simulink model "Product12"  (R2023a)
settings: Solver=VariableStepAuto  StartTime=0.0  StopTime=10.0  RelTol=1e-3
settings Model: Creator=Egypt_Laptop  LastModifiedBy=Egypt_Laptop

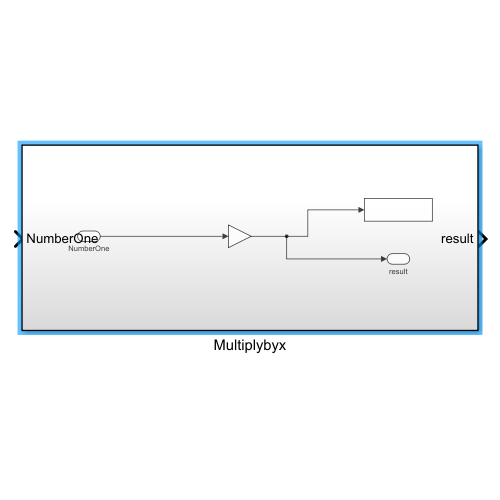
[thumbnail: Simulink's stored preview of the top-level diagram]
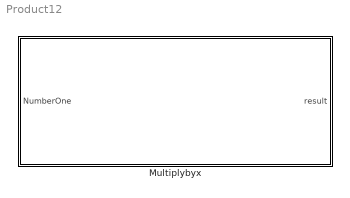
== system Product12 ==
  Multiplybyx : Subsystem

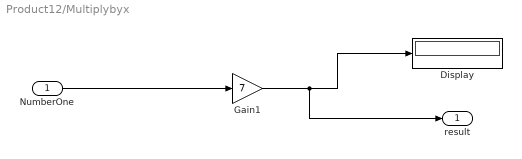
== system Product12/Multiplybyx ==
  NumberOne : Inport
  Display : Display
  Gain1 : Gain  Gain=7
  result : Outport
  wires:
  NumberOne/1 -> Gain1/1
  Gain1/1 -> result/1, Display/1
